simulink model "FOC_sensored"  (R2026a)
settings: Solver=VariableStepAuto  StopTime=3  MaxStep=1e-4  RelTol=1e-4
undefined symbols (not defined in the file): Encoder_resolution, G_filt_back_den_current, G_filt_back_num_current, G_filt_cont_den_current, G_filt_cont_num_current, G_filt_disc_emu_back_den_current, G_filt_disc_emu_back_num_current, G_filt_disc_emu_forw_den_current, G_filt_disc_emu_forw_num_current, G_filt_forw_den_current, G_filt_forw_num_current, In, J, Kr_cont_current, Kr_cont_speed, Kr_direct_back_current, Kr_direct_forw_current, Ld, Lq, Ls, Mn, nn, pp, Psir, T_speed_feedback, Ti_cont_current, Ti_cont_speed, Ti_direct_back_current, Ti_direct_forw_current, Ts_current, Udc
libraries: fl_lib x43, nesl_utility x37, ee_lib x18, eeTransforms x12, slpidlib x5
(part 2 of 2)

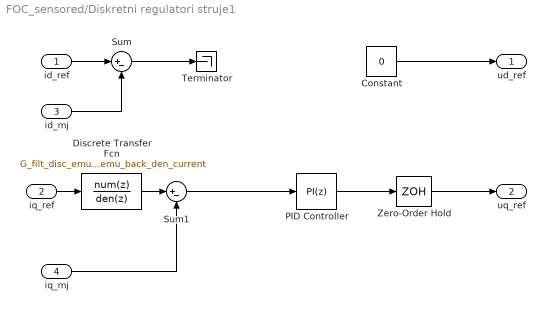
== system FOC_sensored/Diskretni regulatori struje1 ==
  id_ref : Inport
  iq_ref : Inport  Port=2
  id_mj : Inport  Port=3
  iq_mj : Inport  Port=4
  Constant : Constant  Value=0
  Discrete Transfer Fcn : DiscreteTransferFcn  Numerator=G_filt_disc_emu_back_num_current  Denominator=G_filt_disc_emu_back_den_current
  PID Controller : slpidlib/PID Controller  Controller=PI  Form=Ideal  TimeDomain=Discrete-time  UseExternalTs=off  SampleTime=-1  IntegratorMethod=Backward Euler  FilterMethod=Forward Euler  ControllerParametersSource=internal  P=Kr_cont_current  I=1/Ti_cont_current  UseKiTs=off  D=0  UseExternalDerivativeSource=off  N=100  UseFilter=on  TunerSelectOption=Transfer Function Based (PID Tuner App)  InitialConditionSource=internal  InitialConditionForIntegrator=0  InitialConditionForFilter=0  DifferentiatorICPrevScaledInput=0  ExternalReset=none  TrackingMode=off  Kt=1  LimitOutput=off  SatLimitsSource=internal  UpperSaturationLimit=inf  LowerSaturationLimit=-inf  LinearizeAsGain=on  AntiWindupMode=none  Kb=1  LimitIntegrator=off  UpperIntegratorSaturationLimit=inf  LowerIntegratorSaturationLimit=-inf  POutMin=[]  POutMax=[]  IOutMin=[]  IOutMax=[]  DOutMin=[]  DOutMax=[]  NOutMin=[]  NOutMax=[]  SumOutMin=[]  SumOutMax=[]  SaturationOutMin=[]  SaturationOutMax=[]  PParamMin=[]  PParamMax=[]  IParamMin=[]  IParamMax=[]  DParamMin=[]  DParamMax=[]  NParamMin=[]  NParamMax=[]  KbParamMin=[]  KbParamMax=[]  KtParamMin=[]  KtParamMax=[]  KbOutMin=[]  KbOutMax=[]  KtOutMin=[]  KtOutMax=[]  IntegratorOutMin=[]  IntegratorOutMax=[]  FilterOutMin=[]  FilterOutMax=[]  SumI1OutMin=[]  SumI1OutMax=[]  SumI2OutMin=[]  SumI2OutMax=[]  SumI3OutMin=[]  SumI3OutMax=[]  SumI4OutMin=[]  SumI4OutMax=[]  SumDOutMin=[]  SumDOutMax=[]  DifferentiatorOutMin=[]  DifferentiatorOutMax=[]  FilterDiffOutCoefMin=[]  FilterDiffOutCoefMax=[]  ReciprocalOutMin=[]  ReciprocalOutMax=[]  SumDenOutMin=[]  SumDenOutMax=[]  SumNumOutMin=[]  SumNumOutMax=[]  DivideOutMin=[]  DivideOutMax=[]  UdiffTsProdOutMin=[]  UdiffTsProdOutMax=[]  NTsProdOutMin=[]  NTsProdOutMax=[]  UintegralTsProdOutMin=[]  UintegralTsProdOutMax=[]  UngainTsProdOutMin=[]  UngainTsProdOutMax=[]  ClampingZeroOutDataTypeStr=Inherit: Inherit via back propagation  ClampingZeroOutMin=[]  ClampingZeroOutMax=[]  FilterDenConstantOutDataTypeStr=Inherit: Inherit via back propagation  FilterDenConstantOutMin=[]  FilterDenConstantOutMax=[]  PCopyOutDataTypeStr=Inherit: Inherit via back propagation  PCopyOutMin=[]  PCopyOutMax=[]  NCopyOutDataTypeStr=Inherit: Inherit via back propagation  NCopyOutMin=[]  NCopyOutMax=[]  IntegratorContinuousStateAttributes=''  IntegratorStateMustResolveToSignalObject=off  IntegratorRTWStateStorageClass=Auto  FilterContinuousStateAttributes=''  FilterStateMustResolveToSignalObject=off  FilterRTWStateStorageClass=Auto  ParallelPVariant=Passthrough  IdealPVariant=InternalParameters  IVariant=InternalParameters  DVariant=Disabled  IntegratorVariant=Discrete  SatVariant=Disabled  AWVariant=Passthrough  PCopyVariant=Disabled  TRVariant=Disabled  FdbkBlocksVariant=Forward  IdealPFdbkVariant=Disabled  SatFdbkVariant=Disabled  DerivativeFilterVariant=Disabled  NVariant=Disabled  NCopyVariant=Disabled_SignalSpec  FilterICVariant=Disabled  IntegratorICVariant=InternalICs  ExternalResetVariant=Disabled  TRSumVariant=Passthrough  SumFdbkVariant=Disabled  SumVariant=Sum_PI  TsampFilterVariant=InternalTs  TsampNgainVariant=Passthrough  TsampIntegralVariant=Disabled_SignalSpec  ExternalSaturationOutDataTypeStr=Inherit: Same as second input  DerivativeSourceVariant=Disabled  PreIntVariant=InternalPreInt
  Sum : Sum  Inputs=|+-
  Sum1 : Sum  Inputs=|+-
  Terminator : Terminator
  Zero-Order Hold : ZeroOrderHold  SampleTime=Ts_current
  ud_ref : Outport
  uq_ref : Outport  Port=2
  wires:
  iq_mj/1 -> Sum1/2
  Zero-Order Hold/1 -> uq_ref/1
  Sum1/1 -> PID Controller/1
  iq_ref/1 -> Discrete Transfer Fcn/1
  Discrete Transfer Fcn/1 -> Sum1/1
  PID Controller/1 -> Zero-Order Hold/1
  Sum/1 -> Terminator/1
  id_mj/1 -> Sum/2
  id_ref/1 -> Sum/1
  Constant/1 -> ud_ref/1

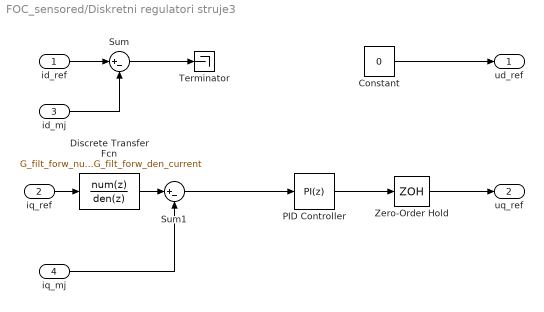
== system FOC_sensored/Diskretni regulatori struje3 ==
  id_ref : Inport
  iq_ref : Inport  Port=2
  id_mj : Inport  Port=3
  iq_mj : Inport  Port=4
  Constant : Constant  Value=0
  Discrete Transfer Fcn : DiscreteTransferFcn  Numerator=G_filt_forw_num_current  Denominator=G_filt_forw_den_current
  PID Controller : slpidlib/PID Controller  Controller=PI  Form=Ideal  TimeDomain=Discrete-time  UseExternalTs=off  SampleTime=-1  IntegratorMethod=Forward Euler  FilterMethod=Forward Euler  ControllerParametersSource=internal  P=Kr_direct_forw_current  I=1/Ti_direct_forw_current  UseKiTs=off  D=0  UseExternalDerivativeSource=off  N=100  UseFilter=on  TunerSelectOption=Transfer Function Based (PID Tuner App)  InitialConditionSource=internal  InitialConditionForIntegrator=0  InitialConditionForFilter=0  DifferentiatorICPrevScaledInput=0  ExternalReset=none  TrackingMode=off  Kt=1  LimitOutput=off  SatLimitsSource=internal  UpperSaturationLimit=inf  LowerSaturationLimit=-inf  LinearizeAsGain=on  AntiWindupMode=none  Kb=1  LimitIntegrator=off  UpperIntegratorSaturationLimit=inf  LowerIntegratorSaturationLimit=-inf  POutMin=[]  POutMax=[]  IOutMin=[]  IOutMax=[]  DOutMin=[]  DOutMax=[]  NOutMin=[]  NOutMax=[]  SumOutMin=[]  SumOutMax=[]  SaturationOutMin=[]  SaturationOutMax=[]  PParamMin=[]  PParamMax=[]  IParamMin=[]  IParamMax=[]  DParamMin=[]  DParamMax=[]  NParamMin=[]  NParamMax=[]  KbParamMin=[]  KbParamMax=[]  KtParamMin=[]  KtParamMax=[]  KbOutMin=[]  KbOutMax=[]  KtOutMin=[]  KtOutMax=[]  IntegratorOutMin=[]  IntegratorOutMax=[]  FilterOutMin=[]  FilterOutMax=[]  SumI1OutMin=[]  SumI1OutMax=[]  SumI2OutMin=[]  SumI2OutMax=[]  SumI3OutMin=[]  SumI3OutMax=[]  SumI4OutMin=[]  SumI4OutMax=[]  SumDOutMin=[]  SumDOutMax=[]  DifferentiatorOutMin=[]  DifferentiatorOutMax=[]  FilterDiffOutCoefMin=[]  FilterDiffOutCoefMax=[]  ReciprocalOutMin=[]  ReciprocalOutMax=[]  SumDenOutMin=[]  SumDenOutMax=[]  SumNumOutMin=[]  SumNumOutMax=[]  DivideOutMin=[]  DivideOutMax=[]  UdiffTsProdOutMin=[]  UdiffTsProdOutMax=[]  NTsProdOutMin=[]  NTsProdOutMax=[]  UintegralTsProdOutMin=[]  UintegralTsProdOutMax=[]  UngainTsProdOutMin=[]  UngainTsProdOutMax=[]  ClampingZeroOutDataTypeStr=Inherit: Inherit via back propagation  ClampingZeroOutMin=[]  ClampingZeroOutMax=[]  FilterDenConstantOutDataTypeStr=Inherit: Inherit via back propagation  FilterDenConstantOutMin=[]  FilterDenConstantOutMax=[]  PCopyOutDataTypeStr=Inherit: Inherit via back propagation  PCopyOutMin=[]  PCopyOutMax=[]  NCopyOutDataTypeStr=Inherit: Inherit via back propagation  NCopyOutMin=[]  NCopyOutMax=[]  IntegratorContinuousStateAttributes=''  IntegratorStateMustResolveToSignalObject=off  IntegratorRTWStateStorageClass=Auto  FilterContinuousStateAttributes=''  FilterStateMustResolveToSignalObject=off  FilterRTWStateStorageClass=Auto  ParallelPVariant=Passthrough  IdealPVariant=InternalParameters  IVariant=InternalParameters  DVariant=Disabled  IntegratorVariant=Discrete  SatVariant=Disabled  AWVariant=Passthrough  PCopyVariant=Disabled  TRVariant=Disabled  FdbkBlocksVariant=Forward  IdealPFdbkVariant=Disabled  SatFdbkVariant=Disabled  DerivativeFilterVariant=Disabled  NVariant=Disabled  NCopyVariant=Disabled_SignalSpec  FilterICVariant=Disabled  IntegratorICVariant=InternalICs  ExternalResetVariant=Disabled  TRSumVariant=Passthrough  SumFdbkVariant=Disabled  SumVariant=Sum_PI  TsampFilterVariant=InternalTs  TsampNgainVariant=Passthrough  TsampIntegralVariant=Disabled_SignalSpec  ExternalSaturationOutDataTypeStr=Inherit: Same as second input  DerivativeSourceVariant=Disabled  PreIntVariant=InternalPreInt
  Sum : Sum  Inputs=|+-
  Sum1 : Sum  Inputs=|+-
  Terminator : Terminator
  Zero-Order Hold : ZeroOrderHold  SampleTime=Ts_current
  ud_ref : Outport
  uq_ref : Outport  Port=2
  wires:
  iq_mj/1 -> Sum1/2
  Zero-Order Hold/1 -> uq_ref/1
  Sum1/1 -> PID Controller/1
  iq_ref/1 -> Discrete Transfer Fcn/1
  Discrete Transfer Fcn/1 -> Sum1/1
  PID Controller/1 -> Zero-Order Hold/1
  Sum/1 -> Terminator/1
  id_mj/1 -> Sum/2
  id_ref/1 -> Sum/1
  Constant/1 -> ud_ref/1

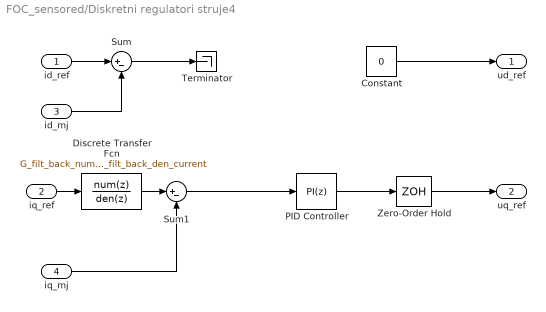
== system FOC_sensored/Diskretni regulatori struje4 ==
  id_ref : Inport
  iq_ref : Inport  Port=2
  id_mj : Inport  Port=3
  iq_mj : Inport  Port=4
  Constant : Constant  Value=0
  Discrete Transfer Fcn : DiscreteTransferFcn  Numerator=G_filt_back_num_current  Denominator=G_filt_back_den_current
  PID Controller : slpidlib/PID Controller  Controller=PI  Form=Ideal  TimeDomain=Discrete-time  UseExternalTs=off  SampleTime=-1  IntegratorMethod=Backward Euler  FilterMethod=Forward Euler  ControllerParametersSource=internal  P=Kr_direct_back_current  I=1/Ti_direct_back_current  UseKiTs=off  D=0  UseExternalDerivativeSource=off  N=100  UseFilter=on  TunerSelectOption=Transfer Function Based (PID Tuner App)  InitialConditionSource=internal  InitialConditionForIntegrator=0  InitialConditionForFilter=0  DifferentiatorICPrevScaledInput=0  ExternalReset=none  TrackingMode=off  Kt=1  LimitOutput=off  SatLimitsSource=internal  UpperSaturationLimit=inf  LowerSaturationLimit=-inf  LinearizeAsGain=on  AntiWindupMode=none  Kb=1  LimitIntegrator=off  UpperIntegratorSaturationLimit=inf  LowerIntegratorSaturationLimit=-inf  POutMin=[]  POutMax=[]  IOutMin=[]  IOutMax=[]  DOutMin=[]  DOutMax=[]  NOutMin=[]  NOutMax=[]  SumOutMin=[]  SumOutMax=[]  SaturationOutMin=[]  SaturationOutMax=[]  PParamMin=[]  PParamMax=[]  IParamMin=[]  IParamMax=[]  DParamMin=[]  DParamMax=[]  NParamMin=[]  NParamMax=[]  KbParamMin=[]  KbParamMax=[]  KtParamMin=[]  KtParamMax=[]  KbOutMin=[]  KbOutMax=[]  KtOutMin=[]  KtOutMax=[]  IntegratorOutMin=[]  IntegratorOutMax=[]  FilterOutMin=[]  FilterOutMax=[]  SumI1OutMin=[]  SumI1OutMax=[]  SumI2OutMin=[]  SumI2OutMax=[]  SumI3OutMin=[]  SumI3OutMax=[]  SumI4OutMin=[]  SumI4OutMax=[]  SumDOutMin=[]  SumDOutMax=[]  DifferentiatorOutMin=[]  DifferentiatorOutMax=[]  FilterDiffOutCoefMin=[]  FilterDiffOutCoefMax=[]  ReciprocalOutMin=[]  ReciprocalOutMax=[]  SumDenOutMin=[]  SumDenOutMax=[]  SumNumOutMin=[]  SumNumOutMax=[]  DivideOutMin=[]  DivideOutMax=[]  UdiffTsProdOutMin=[]  UdiffTsProdOutMax=[]  NTsProdOutMin=[]  NTsProdOutMax=[]  UintegralTsProdOutMin=[]  UintegralTsProdOutMax=[]  UngainTsProdOutMin=[]  UngainTsProdOutMax=[]  ClampingZeroOutDataTypeStr=Inherit: Inherit via back propagation  ClampingZeroOutMin=[]  ClampingZeroOutMax=[]  FilterDenConstantOutDataTypeStr=Inherit: Inherit via back propagation  FilterDenConstantOutMin=[]  FilterDenConstantOutMax=[]  PCopyOutDataTypeStr=Inherit: Inherit via back propagation  PCopyOutMin=[]  PCopyOutMax=[]  NCopyOutDataTypeStr=Inherit: Inherit via back propagation  NCopyOutMin=[]  NCopyOutMax=[]  IntegratorContinuousStateAttributes=''  IntegratorStateMustResolveToSignalObject=off  IntegratorRTWStateStorageClass=Auto  FilterContinuousStateAttributes=''  FilterStateMustResolveToSignalObject=off  FilterRTWStateStorageClass=Auto  ParallelPVariant=Passthrough  IdealPVariant=InternalParameters  IVariant=InternalParameters  DVariant=Disabled  IntegratorVariant=Discrete  SatVariant=Disabled  AWVariant=Passthrough  PCopyVariant=Disabled  TRVariant=Disabled  FdbkBlocksVariant=Forward  IdealPFdbkVariant=Disabled  SatFdbkVariant=Disabled  DerivativeFilterVariant=Disabled  NVariant=Disabled  NCopyVariant=Disabled_SignalSpec  FilterICVariant=Disabled  IntegratorICVariant=InternalICs  ExternalResetVariant=Disabled  TRSumVariant=Passthrough  SumFdbkVariant=Disabled  SumVariant=Sum_PI  TsampFilterVariant=InternalTs  TsampNgainVariant=Passthrough  TsampIntegralVariant=Disabled_SignalSpec  ExternalSaturationOutDataTypeStr=Inherit: Same as second input  DerivativeSourceVariant=Disabled  PreIntVariant=InternalPreInt
  Sum : Sum  Inputs=|+-
  Sum1 : Sum  Inputs=|+-
  Terminator : Terminator
  Zero-Order Hold : ZeroOrderHold  SampleTime=Ts_current
  ud_ref : Outport
  uq_ref : Outport  Port=2
  wires:
  Sum/1 -> Terminator/1
  id_ref/1 -> Sum/1
  Constant/1 -> ud_ref/1
  Sum1/1 -> PID Controller/1
  id_mj/1 -> Sum/2
  iq_mj/1 -> Sum1/2
  Zero-Order Hold/1 -> uq_ref/1
  PID Controller/1 -> Zero-Order Hold/1
  iq_ref/1 -> Discrete Transfer Fcn/1
  Discrete Transfer Fcn/1 -> Sum1/1

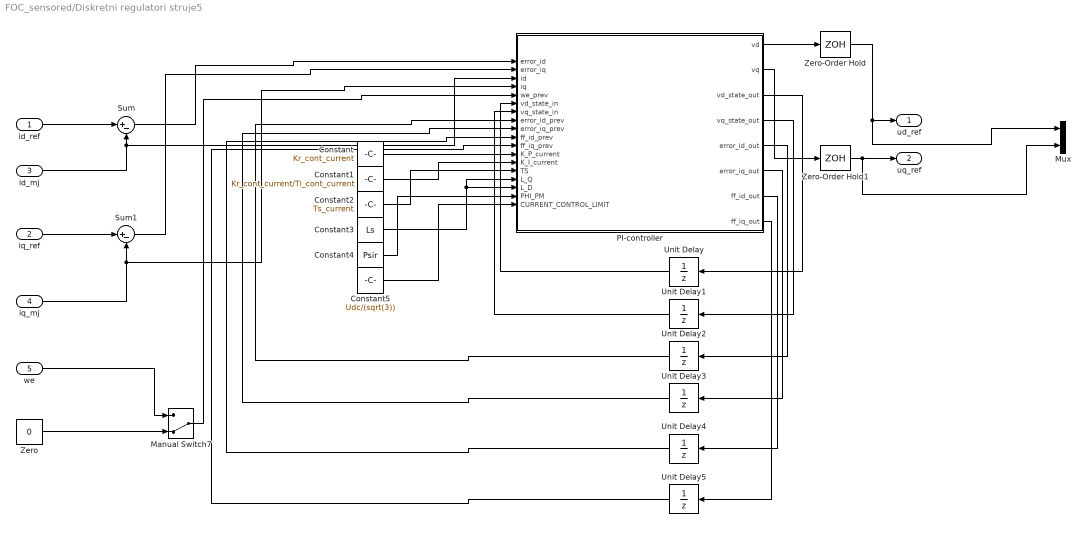
== system FOC_sensored/Diskretni regulatori struje5 ==
  id_ref : Inport
  iq_ref : Inport  Port=2
  id_mj : Inport  Port=3
  iq_mj : Inport  Port=4
  we : Inport  Port=5
  Constant : Constant  Value=Kr_cont_current  SampleTime=Ts_current
  Constant1 : Constant  Value=Kr_cont_current/Ti_cont_current  SampleTime=Ts_current
  Constant2 : Constant  Value=Ts_current  SampleTime=Ts_current
  Constant3 : Constant  Value=Ls  SampleTime=Ts_current
  Constant4 : Constant  Value=Psir  SampleTime=Ts_current
  Constant5 : Constant  Value=Udc/(sqrt(3))  SampleTime=Ts_current
  Manual Switch7 : ManualSwitch  CurrentSetting=0
  Mux : Mux  Inputs=2
  PI-controller : MATLAB Function  TreatAsAtomicUnit=on
  Sum : Sum  Inputs=|+-
  Sum1 : Sum  Inputs=|+-
  Unit Delay{,1..5} (6 alike) : UnitDelay  SampleTime=Ts_current
  Zero : Constant  Value=0  OutDataTypeStr=Inherit: Inherit via back propagation
  Zero-Order Hold : ZeroOrderHold  SampleTime=Ts_current
  Zero-Order Hold1 : ZeroOrderHold  SampleTime=Ts_current
  ud_ref : Outport
  uq_ref : Outport  Port=2
  wires:
  id_ref/1 -> Sum/1
  iq_ref/1 -> Sum1/1
  Sum/1 -> PI-controller/1(error_id)
  Sum1/1 -> PI-controller/2(error_iq)
  id_mj/1 -> Sum/2, PI-controller/3(id)
  iq_mj/1 -> PI-controller/4(iq), Sum1/2
  PI-controller/3(vd_state_out) -> Unit Delay/1
  PI-controller/4(vq_state_out) -> Unit Delay1/1
  PI-controller/5(error_id_out) -> Unit Delay2/1
  PI-controller/6(error_iq_out) -> Unit Delay3/1
  Unit Delay/1 -> PI-controller/6(vd_state_in)
  Unit Delay1/1 -> PI-controller/7(vq_state_in)
  Unit Delay2/1 -> PI-controller/8(error_id_prev)
  Unit Delay3/1 -> PI-controller/9(error_iq_prev)
  PI-controller/1(vd) -> Zero-Order Hold/1
  PI-controller/2(vq) -> Zero-Order Hold1/1
  Zero-Order Hold/1 -> Mux/1, ud_ref/1
  Zero-Order Hold1/1 -> Mux/2, uq_ref/1
  PI-controller/7(ff_id_out) -> Unit Delay4/1
  PI-controller/8(ff_iq_out) -> Unit Delay5/1
  Unit Delay4/1 -> PI-controller/10(ff_id_prev)
  Unit Delay5/1 -> PI-controller/11(ff_iq_prev)
  Zero/1 -> Manual Switch7/2
  Manual Switch7/1 -> PI-controller/5(we_prev)
  we/1 -> Manual Switch7/1
  Constant/1 -> PI-controller/12(K_P_current)
  Constant1/1 -> PI-controller/13(K_I_current)
  Constant2/1 -> PI-controller/14(TS)
  Constant3/1 -> PI-controller/16(L_D), PI-controller/15(L_Q)
  Constant4/1 -> PI-controller/17(PHI_PM)
  Constant5/1 -> PI-controller/18(CURRENT_CONTROL_LIMIT)

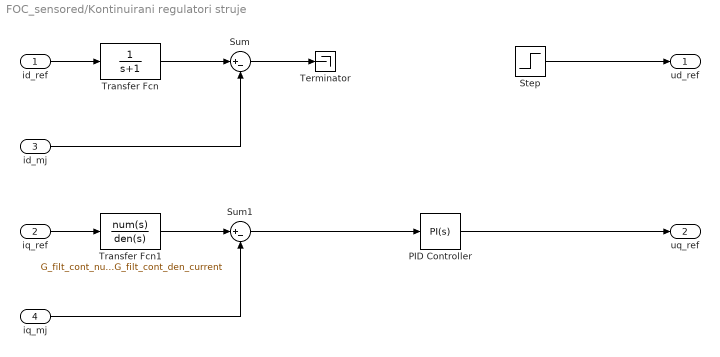
== system FOC_sensored/Kontinuirani regulatori struje ==
  id_ref : Inport
  iq_ref : Inport  Port=2
  id_mj : Inport  Port=3
  iq_mj : Inport  Port=4
  PID Controller : slpidlib/PID Controller  Controller=PI  Form=Ideal  TimeDomain=Continuous-time  UseExternalTs=off  SampleTime=-1  IntegratorMethod=Forward Euler  FilterMethod=Forward Euler  ControllerParametersSource=internal  P=Kr_cont_current  I=1/Ti_cont_current  UseKiTs=off  D=0  UseExternalDerivativeSource=off  N=100  UseFilter=on  TunerSelectOption=Transfer Function Based (PID Tuner App)  InitialConditionSource=internal  InitialConditionForIntegrator=0  InitialConditionForFilter=0  DifferentiatorICPrevScaledInput=0  ExternalReset=none  TrackingMode=off  Kt=1  LimitOutput=off  SatLimitsSource=internal  UpperSaturationLimit=inf  LowerSaturationLimit=-inf  LinearizeAsGain=on  AntiWindupMode=none  Kb=1  LimitIntegrator=off  UpperIntegratorSaturationLimit=inf  LowerIntegratorSaturationLimit=-inf  POutMin=[]  POutMax=[]  IOutMin=[]  IOutMax=[]  DOutMin=[]  DOutMax=[]  NOutMin=[]  NOutMax=[]  SumOutMin=[]  SumOutMax=[]  SaturationOutMin=[]  SaturationOutMax=[]  PParamMin=[]  PParamMax=[]  IParamMin=[]  IParamMax=[]  DParamMin=[]  DParamMax=[]  NParamMin=[]  NParamMax=[]  KbParamMin=[]  KbParamMax=[]  KtParamMin=[]  KtParamMax=[]  KbOutMin=[]  KbOutMax=[]  KtOutMin=[]  KtOutMax=[]  IntegratorOutMin=[]  IntegratorOutMax=[]  FilterOutMin=[]  FilterOutMax=[]  SumI1OutMin=[]  SumI1OutMax=[]  SumI2OutMin=[]  SumI2OutMax=[]  SumI3OutMin=[]  SumI3OutMax=[]  SumI4OutMin=[]  SumI4OutMax=[]  SumDOutMin=[]  SumDOutMax=[]  DifferentiatorOutMin=[]  DifferentiatorOutMax=[]  FilterDiffOutCoefMin=[]  FilterDiffOutCoefMax=[]  ReciprocalOutMin=[]  ReciprocalOutMax=[]  SumDenOutMin=[]  SumDenOutMax=[]  SumNumOutMin=[]  SumNumOutMax=[]  DivideOutMin=[]  DivideOutMax=[]  UdiffTsProdOutMin=[]  UdiffTsProdOutMax=[]  NTsProdOutMin=[]  NTsProdOutMax=[]  UintegralTsProdOutMin=[]  UintegralTsProdOutMax=[]  UngainTsProdOutMin=[]  UngainTsProdOutMax=[]  ClampingZeroOutDataTypeStr=Inherit: Inherit via back propagation  ClampingZeroOutMin=[]  ClampingZeroOutMax=[]  FilterDenConstantOutDataTypeStr=Inherit: Inherit via back propagation  FilterDenConstantOutMin=[]  FilterDenConstantOutMax=[]  PCopyOutDataTypeStr=Inherit: Inherit via back propagation  PCopyOutMin=[]  PCopyOutMax=[]  NCopyOutDataTypeStr=Inherit: Inherit via back propagation  NCopyOutMin=[]  NCopyOutMax=[]  IntegratorContinuousStateAttributes=''  IntegratorStateMustResolveToSignalObject=off  IntegratorRTWStateStorageClass=Auto  FilterContinuousStateAttributes=''  FilterStateMustResolveToSignalObject=off  FilterRTWStateStorageClass=Auto  ParallelPVariant=Passthrough  IdealPVariant=InternalParameters  IVariant=InternalParameters  DVariant=Disabled  IntegratorVariant=Continuous  SatVariant=Disabled  AWVariant=Passthrough  PCopyVariant=Disabled  TRVariant=Disabled  FdbkBlocksVariant=Forward  IdealPFdbkVariant=Disabled  SatFdbkVariant=Disabled  DerivativeFilterVariant=Disabled  NVariant=Disabled  NCopyVariant=Disabled_SignalSpec  FilterICVariant=Disabled  IntegratorICVariant=InternalICs  ExternalResetVariant=Disabled  TRSumVariant=Passthrough  SumFdbkVariant=Disabled  SumVariant=Sum_PI  TsampFilterVariant=InternalTs  TsampNgainVariant=Passthrough  TsampIntegralVariant=Disabled_SignalSpec  ExternalSaturationOutDataTypeStr=Inherit: Same as second input  DerivativeSourceVariant=Disabled  PreIntVariant=InternalPreInt
  Step : Step  FinalValue=0  SampleTime=0
  Sum : Sum  Inputs=|+-
  Sum1 : Sum  Inputs=|+-
  Terminator : Terminator
  Transfer Fcn : TransferFcn  Denominator=[1 1]
  Transfer Fcn1 : TransferFcn  Numerator=G_filt_cont_num_current  Denominator=G_filt_cont_den_current
  ud_ref : Outport
  uq_ref : Outport  Port=2
  wires:
  id_ref/1 -> Transfer Fcn/1
  Transfer Fcn/1 -> Sum/1
  id_mj/1 -> Sum/2
  iq_ref/1 -> Transfer Fcn1/1
  Transfer Fcn1/1 -> Sum1/1
  iq_mj/1 -> Sum1/2
  Sum1/1 -> PID Controller/1
  PID Controller/1 -> uq_ref/1
  Sum/1 -> Terminator/1
  Step/1 -> ud_ref/1

== system FOC_sensored/Mjerenje momenta ==
  PS-Simulink Converter3 : nesl_utility/PS-Simulink Converter  PhysicalDomain=network_engine_domain  SubClassName=ps_output  LeftPortType=input  RightPortType=output  PseudoPeriodic=off  Frequencies=[]  VectorFormat=1-D array  Unit=N*m  AffineConversion=off
  Torque Sensor : fl_lib/Mechanical/Mechanical Sensors/Ideal Torque Sensor
  R : PMIOPort  Side=Left
  C : PMIOPort  Port=2  Side=Right
  Output : Outport
  wires:
  PS-Simulink Converter3/1 -> Output/1
  connections:
  Torque Sensor/RConn1 -- C/RConn1
  Torque Sensor/RConn2 -- PS-Simulink Converter3/LConn1
  Torque Sensor/LConn1 -- R/RConn1

== system FOC_sensored/Mjerenje momenta1 ==
  PS-Simulink Converter3 : nesl_utility/PS-Simulink Converter  PhysicalDomain=network_engine_domain  SubClassName=ps_output  LeftPortType=input  RightPortType=output  PseudoPeriodic=off  Frequencies=[]  VectorFormat=1-D array  Unit=N*m  AffineConversion=off
  Torque Sensor : fl_lib/Mechanical/Mechanical Sensors/Ideal Torque Sensor
  R : PMIOPort  Side=Left
  C : PMIOPort  Port=2  Side=Right
  Output : Outport
  wires:
  PS-Simulink Converter3/1 -> Output/1
  connections:
  Torque Sensor/RConn1 -- C/RConn1
  Torque Sensor/RConn2 -- PS-Simulink Converter3/LConn1
  Torque Sensor/LConn1 -- R/RConn1

== system FOC_sensored/Mjerenje momenta2 ==
  PS-Simulink Converter3 : nesl_utility/PS-Simulink Converter  PhysicalDomain=network_engine_domain  SubClassName=ps_output  LeftPortType=input  RightPortType=output  PseudoPeriodic=off  Frequencies=[]  VectorFormat=1-D array  Unit=N*m  AffineConversion=off
  Torque Sensor : fl_lib/Mechanical/Mechanical Sensors/Ideal Torque Sensor
  R : PMIOPort  Side=Left
  C : PMIOPort  Port=2  Side=Right
  Output : Outport
  wires:
  PS-Simulink Converter3/1 -> Output/1
  connections:
  Torque Sensor/RConn1 -- C/RConn1
  Torque Sensor/RConn2 -- PS-Simulink Converter3/LConn1
  Torque Sensor/LConn1 -- R/RConn1

== system FOC_sensored/Mjerenje momenta4 ==
  PS-Simulink Converter3 : nesl_utility/PS-Simulink Converter  PhysicalDomain=network_engine_domain  SubClassName=ps_output  LeftPortType=input  RightPortType=output  PseudoPeriodic=off  Frequencies=[]  VectorFormat=1-D array  Unit=N*m  AffineConversion=off
  Torque Sensor : fl_lib/Mechanical/Mechanical Sensors/Ideal Torque Sensor
  R : PMIOPort  Side=Left
  C : PMIOPort  Port=2  Side=Right
  Output : Outport
  wires:
  PS-Simulink Converter3/1 -> Output/1
  connections:
  Torque Sensor/RConn1 -- C/RConn1
  Torque Sensor/RConn2 -- PS-Simulink Converter3/LConn1
  Torque Sensor/LConn1 -- R/RConn1

== system FOC_sensored/Mjerenje momenta5 ==
  PS-Simulink Converter3 : nesl_utility/PS-Simulink Converter  PhysicalDomain=network_engine_domain  SubClassName=ps_output  LeftPortType=input  RightPortType=output  PseudoPeriodic=off  Frequencies=[]  VectorFormat=1-D array  Unit=N*m  AffineConversion=off
  Torque Sensor : fl_lib/Mechanical/Mechanical Sensors/Ideal Torque Sensor
  R : PMIOPort  Side=Left
  C : PMIOPort  Port=2  Side=Right
  Output : Outport
  wires:
  PS-Simulink Converter3/1 -> Output/1
  connections:
  Torque Sensor/RConn1 -- C/RConn1
  Torque Sensor/RConn2 -- PS-Simulink Converter3/LConn1
  Torque Sensor/LConn1 -- R/RConn1

== system FOC_sensored/Mjerenje momenta6 ==
  PS-Simulink Converter3 : nesl_utility/PS-Simulink Converter  PhysicalDomain=network_engine_domain  SubClassName=ps_output  LeftPortType=input  RightPortType=output  PseudoPeriodic=off  Frequencies=[]  VectorFormat=1-D array  Unit=N*m  AffineConversion=off
  Torque Sensor : fl_lib/Mechanical/Mechanical Sensors/Ideal Torque Sensor
  R : PMIOPort  Side=Left
  C : PMIOPort  Port=2  Side=Right
  Output : Outport
  wires:
  PS-Simulink Converter3/1 -> Output/1
  connections:
  Torque Sensor/RConn1 -- C/RConn1
  Torque Sensor/RConn2 -- PS-Simulink Converter3/LConn1
  Torque Sensor/LConn1 -- R/RConn1

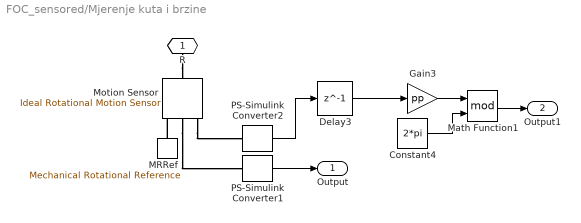
== system FOC_sensored/Mjerenje kuta i brzine ==
  Constant4 : Constant  Value=2*pi
  Delay3 : Delay  DelayLength=1  SampleTime=Ts_current
  Gain3 : Gain  Gain=pp
  MRRef : fl_lib/Mechanical/Rotational Elements/Mechanical Rotational Reference
  Math Function1 : Math  Operator=mod
  Motion Sensor : fl_lib/Mechanical/Mechanical Sensors/Ideal Rotational Motion Sensor  reference=foundation.enum.MeasurementReference.difference  acceleration_port=false  velocity_port=true  position_port=true  wrap_angle=simscape.enum.onoff.off  offset=0 deg
  PS-Simulink Converter1 : nesl_utility/PS-Simulink Converter  PhysicalDomain=network_engine_domain  SubClassName=ps_output  LeftPortType=input  RightPortType=output  PseudoPeriodic=off  Frequencies=[]  VectorFormat=1-D array  Unit=rad/s  AffineConversion=off
  PS-Simulink Converter2 : nesl_utility/PS-Simulink Converter  PhysicalDomain=network_engine_domain  SubClassName=ps_output  LeftPortType=input  RightPortType=output  PseudoPeriodic=off  Frequencies=[]  VectorFormat=1-D array  Unit=rad  AffineConversion=off
  R : PMIOPort  Side=Left
  Output : Outport
  Output1 : Outport  Port=2
  wires:
  PS-Simulink Converter1/1 -> Output/1
  Gain3/1 -> Math Function1/1
  Delay3/1 -> Gain3/1
  Constant4/1 -> Math Function1/2
  Math Function1/1 -> Output1/1
  PS-Simulink Converter2/1 -> Delay3/1
  connections:
  R/RConn1 -- Motion Sensor/LConn1
  Motion Sensor/RConn2 -- PS-Simulink Converter1/LConn1
  MRRef/LConn1 -- Motion Sensor/RConn1
  Motion Sensor/RConn3 -- PS-Simulink Converter2/LConn1

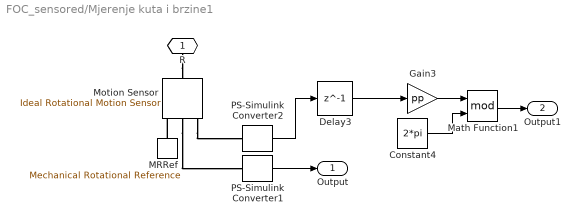
== system FOC_sensored/Mjerenje kuta i brzine1 ==
  Constant4 : Constant  Value=2*pi
  Delay3 : Delay  DelayLength=1  SampleTime=Ts_current
  Gain3 : Gain  Gain=pp
  MRRef : fl_lib/Mechanical/Rotational Elements/Mechanical Rotational Reference
  Math Function1 : Math  Operator=mod
  Motion Sensor : fl_lib/Mechanical/Mechanical Sensors/Ideal Rotational Motion Sensor  reference=foundation.enum.MeasurementReference.difference  acceleration_port=false  velocity_port=true  position_port=true  wrap_angle=simscape.enum.onoff.off  offset=0 deg
  PS-Simulink Converter1 : nesl_utility/PS-Simulink Converter  PhysicalDomain=network_engine_domain  SubClassName=ps_output  LeftPortType=input  RightPortType=output  PseudoPeriodic=off  Frequencies=[]  VectorFormat=1-D array  Unit=rad/s  AffineConversion=off
  PS-Simulink Converter2 : nesl_utility/PS-Simulink Converter  PhysicalDomain=network_engine_domain  SubClassName=ps_output  LeftPortType=input  RightPortType=output  PseudoPeriodic=off  Frequencies=[]  VectorFormat=1-D array  Unit=rad  AffineConversion=off
  R : PMIOPort  Side=Left
  Output : Outport
  Output1 : Outport  Port=2
  wires:
  PS-Simulink Converter1/1 -> Output/1
  Gain3/1 -> Math Function1/1
  Delay3/1 -> Gain3/1
  Constant4/1 -> Math Function1/2
  Math Function1/1 -> Output1/1
  PS-Simulink Converter2/1 -> Delay3/1
  connections:
  R/RConn1 -- Motion Sensor/LConn1
  Motion Sensor/RConn2 -- PS-Simulink Converter1/LConn1
  MRRef/LConn1 -- Motion Sensor/RConn1
  Motion Sensor/RConn3 -- PS-Simulink Converter2/LConn1

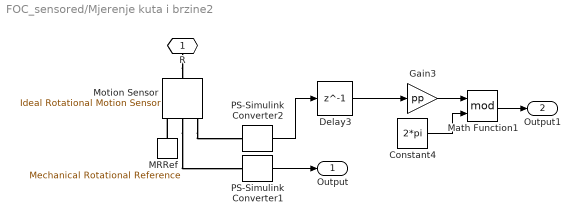
== system FOC_sensored/Mjerenje kuta i brzine2 ==
  Constant4 : Constant  Value=2*pi
  Delay3 : Delay  DelayLength=1  SampleTime=Ts_current
  Gain3 : Gain  Gain=pp
  MRRef : fl_lib/Mechanical/Rotational Elements/Mechanical Rotational Reference
  Math Function1 : Math  Operator=mod
  Motion Sensor : fl_lib/Mechanical/Mechanical Sensors/Ideal Rotational Motion Sensor  reference=foundation.enum.MeasurementReference.difference  acceleration_port=false  velocity_port=true  position_port=true  wrap_angle=simscape.enum.onoff.off  offset=0 deg
  PS-Simulink Converter1 : nesl_utility/PS-Simulink Converter  PhysicalDomain=network_engine_domain  SubClassName=ps_output  LeftPortType=input  RightPortType=output  PseudoPeriodic=off  Frequencies=[]  VectorFormat=1-D array  Unit=rad/s  AffineConversion=off
  PS-Simulink Converter2 : nesl_utility/PS-Simulink Converter  PhysicalDomain=network_engine_domain  SubClassName=ps_output  LeftPortType=input  RightPortType=output  PseudoPeriodic=off  Frequencies=[]  VectorFormat=1-D array  Unit=rad  AffineConversion=off
  R : PMIOPort  Side=Left
  Output : Outport
  Output1 : Outport  Port=2
  wires:
  PS-Simulink Converter1/1 -> Output/1
  Gain3/1 -> Math Function1/1
  Delay3/1 -> Gain3/1
  Constant4/1 -> Math Function1/2
  Math Function1/1 -> Output1/1
  PS-Simulink Converter2/1 -> Delay3/1
  connections:
  R/RConn1 -- Motion Sensor/LConn1
  Motion Sensor/RConn2 -- PS-Simulink Converter1/LConn1
  MRRef/LConn1 -- Motion Sensor/RConn1
  Motion Sensor/RConn3 -- PS-Simulink Converter2/LConn1

== system FOC_sensored/Mjerenje kuta i brzine4 ==
  Constant4 : Constant  Value=2*pi
  Delay3 : Delay  DelayLength=1  SampleTime=Ts_current
  Gain3 : Gain  Gain=pp
  MRRef : fl_lib/Mechanical/Rotational Elements/Mechanical Rotational Reference
  Math Function1 : Math  Operator=mod
  Motion Sensor : fl_lib/Mechanical/Mechanical Sensors/Ideal Rotational Motion Sensor  reference=foundation.enum.MeasurementReference.difference  acceleration_port=false  velocity_port=true  position_port=true  wrap_angle=simscape.enum.onoff.off  offset=0 deg
  PS-Simulink Converter1 : nesl_utility/PS-Simulink Converter  PhysicalDomain=network_engine_domain  SubClassName=ps_output  LeftPortType=input  RightPortType=output  PseudoPeriodic=off  Frequencies=[]  VectorFormat=1-D array  Unit=rad/s  AffineConversion=off
  PS-Simulink Converter2 : nesl_utility/PS-Simulink Converter  PhysicalDomain=network_engine_domain  SubClassName=ps_output  LeftPortType=input  RightPortType=output  PseudoPeriodic=off  Frequencies=[]  VectorFormat=1-D array  Unit=rad  AffineConversion=off
  R : PMIOPort  Side=Left
  Output : Outport
  Output1 : Outport  Port=2
  wires:
  PS-Simulink Converter1/1 -> Output/1
  Gain3/1 -> Math Function1/1
  Delay3/1 -> Gain3/1
  Constant4/1 -> Math Function1/2
  Math Function1/1 -> Output1/1
  PS-Simulink Converter2/1 -> Delay3/1
  connections:
  R/RConn1 -- Motion Sensor/LConn1
  Motion Sensor/RConn2 -- PS-Simulink Converter1/LConn1
  MRRef/LConn1 -- Motion Sensor/RConn1
  Motion Sensor/RConn3 -- PS-Simulink Converter2/LConn1

== system FOC_sensored/Mjerenje kuta i brzine5 ==
  Constant4 : Constant  Value=2*pi
  Delay3 : Delay  DelayLength=1  SampleTime=Ts_current
  Gain3 : Gain  Gain=pp
  MRRef : fl_lib/Mechanical/Rotational Elements/Mechanical Rotational Reference
  Math Function1 : Math  Operator=mod
  Motion Sensor : fl_lib/Mechanical/Mechanical Sensors/Ideal Rotational Motion Sensor  reference=foundation.enum.MeasurementReference.difference  acceleration_port=false  velocity_port=true  position_port=true  wrap_angle=simscape.enum.onoff.off  offset=0 deg
  PS-Simulink Converter1 : nesl_utility/PS-Simulink Converter  PhysicalDomain=network_engine_domain  SubClassName=ps_output  LeftPortType=input  RightPortType=output  PseudoPeriodic=off  Frequencies=[]  VectorFormat=1-D array  Unit=rad/s  AffineConversion=off
  PS-Simulink Converter2 : nesl_utility/PS-Simulink Converter  PhysicalDomain=network_engine_domain  SubClassName=ps_output  LeftPortType=input  RightPortType=output  PseudoPeriodic=off  Frequencies=[]  VectorFormat=1-D array  Unit=rad  AffineConversion=off
  R : PMIOPort  Side=Left
  Output : Outport
  Output1 : Outport  Port=2
  wires:
  PS-Simulink Converter1/1 -> Output/1
  Gain3/1 -> Math Function1/1
  Delay3/1 -> Gain3/1
  Constant4/1 -> Math Function1/2
  Math Function1/1 -> Output1/1
  PS-Simulink Converter2/1 -> Delay3/1
  connections:
  R/RConn1 -- Motion Sensor/LConn1
  Motion Sensor/RConn2 -- PS-Simulink Converter1/LConn1
  MRRef/LConn1 -- Motion Sensor/RConn1
  Motion Sensor/RConn3 -- PS-Simulink Converter2/LConn1

== system FOC_sensored/Mjerenje kuta i brzine6 ==
  Constant4 : Constant  Value=2*pi
  Gain : Gain  Gain=pp
  Gain3 : Gain  Gain=pp
  MRRef : fl_lib/Mechanical/Rotational Elements/Mechanical Rotational Reference
  Math Function1 : Math  Operator=mod
  Motion Sensor : fl_lib/Mechanical/Mechanical Sensors/Ideal Rotational Motion Sensor  reference=foundation.enum.MeasurementReference.difference  acceleration_port=false  velocity_port=true  position_port=true  wrap_angle=simscape.enum.onoff.off  offset=0 deg
  PS-Simulink Converter1 : nesl_utility/PS-Simulink Converter  PhysicalDomain=network_engine_domain  SubClassName=ps_output  LeftPortType=input  RightPortType=output  PseudoPeriodic=off  Frequencies=[]  VectorFormat=1-D array  Unit=rad/s  AffineConversion=off
  PS-Simulink Converter2 : nesl_utility/PS-Simulink Converter  PhysicalDomain=network_engine_domain  SubClassName=ps_output  LeftPortType=input  RightPortType=output  PseudoPeriodic=off  Frequencies=[]  VectorFormat=1-D array  Unit=rad  AffineConversion=off
  R : PMIOPort  Side=Left
  we : Outport
  theta_e : Outport  Port=2
  wires:
  PS-Simulink Converter1/1 -> Gain/1
  Gain/1 -> we/1
  PS-Simulink Converter2/1 -> Gain3/1
  Constant4/1 -> Math Function1/2
  Gain3/1 -> Math Function1/1
  Math Function1/1 -> theta_e/1
  connections:
  R/RConn1 -- Motion Sensor/LConn1
  Motion Sensor/RConn2 -- PS-Simulink Converter1/LConn1
  MRRef/LConn1 -- Motion Sensor/RConn1
  Motion Sensor/RConn3 -- PS-Simulink Converter2/LConn1

== system FOC_sensored/Mjerenje struje ==
  Input : Inport
  Current Sensor : ee_lib/Sensors & Transducers/Current Sensor (Three-Phase)  port_option=ee.enum.threePhasePort.composite
  PS-Simulink Converter : nesl_utility/PS-Simulink Converter  PhysicalDomain=network_engine_domain  SubClassName=ps_output  LeftPortType=input  RightPortType=output  PseudoPeriodic=off  Frequencies=[]  VectorFormat=1-D array  Unit=1  AffineConversion=off
  Park Transform : eeTransforms/Park Transform  AxisAlignment=D-axis  PowerInvariant=off
  ~1 : PMIOPort  Side=Left
  ~2 : PMIOPort  Port=2  Side=Right
  Output : Outport
  wires:
  PS-Simulink Converter/1 -> Park Transform/1
  Park Transform/1 -> Output/1
  Input/1 -> Park Transform/2
  connections:
  Current Sensor/LConn1 -- ~1/RConn1
  PS-Simulink Converter/LConn1 -- Current Sensor/RConn1
  Current Sensor/RConn2 -- ~2/RConn1

== system FOC_sensored/Mjerenje struje1 ==
  Input : Inport
  Current Sensor : ee_lib/Sensors & Transducers/Current Sensor (Three-Phase)  port_option=ee.enum.threePhasePort.composite
  PS-Simulink Converter : nesl_utility/PS-Simulink Converter  PhysicalDomain=network_engine_domain  SubClassName=ps_output  LeftPortType=input  RightPortType=output  PseudoPeriodic=off  Frequencies=[]  VectorFormat=1-D array  Unit=1  AffineConversion=off
  Park Transform : eeTransforms/Park Transform  AxisAlignment=D-axis  PowerInvariant=off
  ~1 : PMIOPort  Side=Left
  ~2 : PMIOPort  Port=2  Side=Right
  Output : Outport
  wires:
  PS-Simulink Converter/1 -> Park Transform/1
  Park Transform/1 -> Output/1
  Input/1 -> Park Transform/2
  connections:
  Current Sensor/LConn1 -- ~1/RConn1
  PS-Simulink Converter/LConn1 -- Current Sensor/RConn1
  Current Sensor/RConn2 -- ~2/RConn1

== system FOC_sensored/Mjerenje struje3 ==
  Input : Inport
  Current Sensor : ee_lib/Sensors & Transducers/Current Sensor (Three-Phase)  port_option=ee.enum.threePhasePort.composite
  PS-Simulink Converter : nesl_utility/PS-Simulink Converter  PhysicalDomain=network_engine_domain  SubClassName=ps_output  LeftPortType=input  RightPortType=output  PseudoPeriodic=off  Frequencies=[]  VectorFormat=1-D array  Unit=1  AffineConversion=off
  Park Transform : eeTransforms/Park Transform  AxisAlignment=D-axis  PowerInvariant=off
  ~1 : PMIOPort  Side=Left
  ~2 : PMIOPort  Port=2  Side=Right
  Output : Outport
  wires:
  PS-Simulink Converter/1 -> Park Transform/1
  Park Transform/1 -> Output/1
  Input/1 -> Park Transform/2
  connections:
  Current Sensor/LConn1 -- ~1/RConn1
  PS-Simulink Converter/LConn1 -- Current Sensor/RConn1
  Current Sensor/RConn2 -- ~2/RConn1

== system FOC_sensored/Mjerenje struje4 ==
  Input : Inport
  Current Sensor : ee_lib/Sensors & Transducers/Current Sensor (Three-Phase)  port_option=ee.enum.threePhasePort.composite
  PS-Simulink Converter : nesl_utility/PS-Simulink Converter  PhysicalDomain=network_engine_domain  SubClassName=ps_output  LeftPortType=input  RightPortType=output  PseudoPeriodic=off  Frequencies=[]  VectorFormat=1-D array  Unit=1  AffineConversion=off
  Park Transform : eeTransforms/Park Transform  AxisAlignment=D-axis  PowerInvariant=off
  ~1 : PMIOPort  Side=Left
  ~2 : PMIOPort  Port=2  Side=Right
  Output : Outport
  wires:
  PS-Simulink Converter/1 -> Park Transform/1
  Park Transform/1 -> Output/1
  Input/1 -> Park Transform/2
  connections:
  Current Sensor/LConn1 -- ~1/RConn1
  PS-Simulink Converter/LConn1 -- Current Sensor/RConn1
  Current Sensor/RConn2 -- ~2/RConn1

== system FOC_sensored/Mjerenje struje5 ==
  Input : Inport
  Current Sensor : ee_lib/Sensors & Transducers/Current Sensor (Three-Phase)  port_option=ee.enum.threePhasePort.composite
  PS-Simulink Converter : nesl_utility/PS-Simulink Converter  PhysicalDomain=network_engine_domain  SubClassName=ps_output  LeftPortType=input  RightPortType=output  PseudoPeriodic=off  Frequencies=[]  VectorFormat=1-D array  Unit=1  AffineConversion=off
  Park Transform : eeTransforms/Park Transform  AxisAlignment=D-axis  PowerInvariant=off
  ~1 : PMIOPort  Side=Left
  ~2 : PMIOPort  Port=2  Side=Right
  Output : Outport
  wires:
  PS-Simulink Converter/1 -> Park Transform/1
  Park Transform/1 -> Output/1
  Input/1 -> Park Transform/2
  connections:
  Current Sensor/LConn1 -- ~1/RConn1
  PS-Simulink Converter/LConn1 -- Current Sensor/RConn1
  Current Sensor/RConn2 -- ~2/RConn1

== system FOC_sensored/Mjerenje struje7 ==
  Input : Inport
  Current Sensor : ee_lib/Sensors & Transducers/Current Sensor (Three-Phase)  port_option=ee.enum.threePhasePort.composite
  PS-Simulink Converter : nesl_utility/PS-Simulink Converter  PhysicalDomain=network_engine_domain  SubClassName=ps_output  LeftPortType=input  RightPortType=output  PseudoPeriodic=off  Frequencies=[]  VectorFormat=1-D array  Unit=1  AffineConversion=off
  Park Transform : eeTransforms/Park Transform  AxisAlignment=D-axis  PowerInvariant=off
  ~1 : PMIOPort  Side=Left
  ~2 : PMIOPort  Port=2  Side=Right
  Output : Outport
  wires:
  PS-Simulink Converter/1 -> Park Transform/1
  Park Transform/1 -> Output/1
  Input/1 -> Park Transform/2
  connections:
  Current Sensor/LConn1 -- ~1/RConn1
  PS-Simulink Converter/LConn1 -- Current Sensor/RConn1
  Current Sensor/RConn2 -- ~2/RConn1

== system FOC_sensored/PWM inverter1 ==
  ud_ref : Inport
  uq_ref : Inport  Port=2
  theta_e_mj : Inport  Port=3
  Constant1 : Constant  Value=0  SampleTime=-1
  Gain : Gain
  Gain1 : Gain
  Mux2 : Mux  Inputs=2
  Mux3 : Mux  Inputs=2
  dq->abc : eeTransforms/Inverse Park Transform  AxisAlignment=D-axis  PowerInvariant=off
  u_abc* : Outport  VectorParamsAs1DForOutWhenUnconnected=off
  wires:
  Constant1/1 -> Mux2/2
  Mux2/1 -> dq->abc/1
  Mux3/1 -> Mux2/1
  theta_e_mj/1 -> dq->abc/2
  ud_ref/1 -> Gain/1
  uq_ref/1 -> Gain1/1
  Gain/1 -> Mux3/1
  Gain1/1 -> Mux3/2
  dq->abc/1 -> u_abc*/1

== system FOC_sensored/PWM inverter2 ==
  ud_ref : Inport
  uq_ref : Inport  Port=2
  theta_e_mj : Inport  Port=3
  Constant1 : Constant  Value=0  SampleTime=-1
  Gain : Gain
  Gain1 : Gain
  Mux2 : Mux  Inputs=2
  Mux3 : Mux  Inputs=2
  Zero-Order Hold1 : ZeroOrderHold  SampleTime=Ts_current
  dq->abc : eeTransforms/Inverse Park Transform  AxisAlignment=D-axis  PowerInvariant=off
  u_abc* : Outport  VectorParamsAs1DForOutWhenUnconnected=off
  wires:
  Constant1/1 -> Mux2/2
  Mux2/1 -> dq->abc/1
  Mux3/1 -> Mux2/1
  theta_e_mj/1 -> dq->abc/2
  dq->abc/1 -> Zero-Order Hold1/1
  ud_ref/1 -> Gain/1
  uq_ref/1 -> Gain1/1
  Gain/1 -> Mux3/1
  Gain1/1 -> Mux3/2
  Zero-Order Hold1/1 -> u_abc*/1

== system FOC_sensored/PWM inverter3 ==
  ud_ref : Inport
  uq_ref : Inport  Port=2
  theta_e_mj : Inport  Port=3
  Constant1 : Constant  Value=0  SampleTime=-1
  Gain : Gain
  Gain1 : Gain
  Mux2 : Mux  Inputs=2
  Mux3 : Mux  Inputs=2
  Zero-Order Hold1 : ZeroOrderHold  SampleTime=Ts_current
  dq->abc : eeTransforms/Inverse Park Transform  AxisAlignment=D-axis  PowerInvariant=off
  u_abc* : Outport  VectorParamsAs1DForOutWhenUnconnected=off
  wires:
  Constant1/1 -> Mux2/2
  Mux2/1 -> dq->abc/1
  Mux3/1 -> Mux2/1
  theta_e_mj/1 -> dq->abc/2
  dq->abc/1 -> Zero-Order Hold1/1
  ud_ref/1 -> Gain/1
  uq_ref/1 -> Gain1/1
  Gain/1 -> Mux3/1
  Gain1/1 -> Mux3/2
  Zero-Order Hold1/1 -> u_abc*/1

== system FOC_sensored/PWM inverter5 ==
  ud_ref : Inport
  uq_ref : Inport  Port=2
  theta_e_mj : Inport  Port=3
  Constant1 : Constant  Value=0  SampleTime=-1
  Gain : Gain
  Gain1 : Gain
  Mux2 : Mux  Inputs=2
  Mux3 : Mux  Inputs=2
  Zero-Order Hold1 : ZeroOrderHold  SampleTime=Ts_current
  dq->abc : eeTransforms/Inverse Park Transform  AxisAlignment=D-axis  PowerInvariant=off
  u_abc* : Outport  VectorParamsAs1DForOutWhenUnconnected=off
  wires:
  Constant1/1 -> Mux2/2
  Mux2/1 -> dq->abc/1
  Mux3/1 -> Mux2/1
  theta_e_mj/1 -> dq->abc/2
  dq->abc/1 -> Zero-Order Hold1/1
  ud_ref/1 -> Gain/1
  uq_ref/1 -> Gain1/1
  Gain/1 -> Mux3/1
  Gain1/1 -> Mux3/2
  Zero-Order Hold1/1 -> u_abc*/1

== system FOC_sensored/PWM inverter6 ==
  ud_ref : Inport
  uq_ref : Inport  Port=2
  theta_e_mj : Inport  Port=3
  Constant1 : Constant  Value=0  SampleTime=-1
  Gain : Gain
  Gain1 : Gain
  Mux2 : Mux  Inputs=2
  Mux3 : Mux  Inputs=2
  Zero-Order Hold1 : ZeroOrderHold  SampleTime=Ts_current
  dq->abc : eeTransforms/Inverse Park Transform  AxisAlignment=D-axis  PowerInvariant=off
  u_abc* : Outport  VectorParamsAs1DForOutWhenUnconnected=off
  wires:
  Constant1/1 -> Mux2/2
  Mux2/1 -> dq->abc/1
  Mux3/1 -> Mux2/1
  theta_e_mj/1 -> dq->abc/2
  dq->abc/1 -> Zero-Order Hold1/1
  ud_ref/1 -> Gain/1
  uq_ref/1 -> Gain1/1
  Gain/1 -> Mux3/1
  Gain1/1 -> Mux3/2
  Zero-Order Hold1/1 -> u_abc*/1

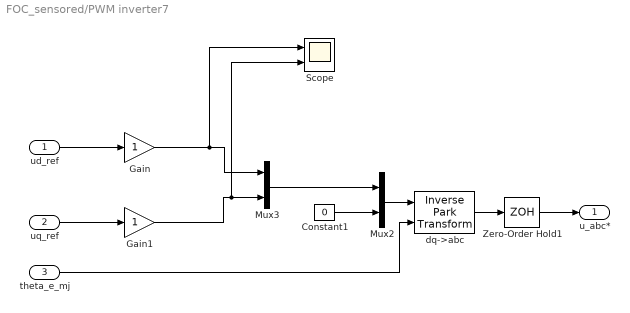
== system FOC_sensored/PWM inverter7 ==
  ud_ref : Inport
  uq_ref : Inport  Port=2
  theta_e_mj : Inport  Port=3
  Constant1 : Constant  Value=0  SampleTime=-1
  Gain : Gain
  Gain1 : Gain
  Mux2 : Mux  Inputs=2
  Mux3 : Mux  Inputs=2
  Scope : Scope  NumInputPorts=2
      settings: ActiveDisplayYMinimum=-5.00439749396322  ActiveDisplayYMaximum=16.069405098335697
  Zero-Order Hold1 : ZeroOrderHold  SampleTime=Ts_current
  dq->abc : eeTransforms/Inverse Park Transform  AxisAlignment=D-axis  PowerInvariant=off
  u_abc* : Outport  VectorParamsAs1DForOutWhenUnconnected=off
  wires:
  Constant1/1 -> Mux2/2
  Mux2/1 -> dq->abc/1
  Mux3/1 -> Mux2/1
  theta_e_mj/1 -> dq->abc/2
  dq->abc/1 -> Zero-Order Hold1/1
  ud_ref/1 -> Gain/1
  uq_ref/1 -> Gain1/1
  Gain/1 -> Scope/1, Mux3/1
  Gain1/1 -> Scope/2, Mux3/2
  Zero-Order Hold1/1 -> u_abc*/1

== matlab function FOC_sensored/Low-Pass Filter Current ==
  data: x input; y output; y_prev input; y_prev_out output; x_prev input; x_prev_out output; fc input; TS input
function [y, y_prev_out, x_prev_out] = fcn(x, y_prev, x_prev, fc, TS)



%% Convert to rad/s
omega_c = 2 * pi * fc;

%% Tustin coefficients
b =  omega_c / (2/TS + omega_c);
a = (omega_c - 2/TS) / (2/TS + omega_c);

%% Output
y = b * (x + x_prev) - a * y_prev;

%% State outputs — two separate scalars
y_prev_out = y;
x_prev_out = x;

end

== matlab function FOC_sensored/Low-Pass Filter Speed Ref ==
  data: x input; y output; y_prev input; y_prev_out output; x_prev input; x_prev_out output; fc input; TS input
function [y, y_prev_out, x_prev_out] = fcn(x, y_prev, x_prev, fc, TS)

%% Convert to rad/s
omega_c = 2 * pi * fc;

%% Tustin coefficients
b =  omega_c / (2/TS + omega_c);
a = (omega_c - 2/TS) / (2/TS + omega_c);

%% Output
y = b * (x + x_prev) - a * y_prev;

%% State outputs — two separate scalars
y_prev_out = y;
x_prev_out = x;

end

== matlab function FOC_sensored/Encoder ==
  data: angle input; theta_e output; omega_e output; angle_prev input; q_angle output; N input; dt input; pole_pairs input
function [theta_e, omega_e, q_angle] = fcn(angle, angle_prev, N, dt, pole_pairs)

%% Quantize current angle (simulate encoder resolution)
raw_count   = angle * (N / (2*pi));
counts      = floor(raw_count + 0.5);
q_angle     = counts * (2*pi / N);

%% Quantize previous angle the same way
raw_count_prev = angle_prev * (N / (2*pi));
counts_prev    = floor(raw_count_prev + 0.5);
q_angle_prev   = counts_prev * (2*pi / N);

%% Mechanical angular velocity (handle wrap-around)
delta = q_angle - q_angle_prev;

% Unwrap: if jump > pi, crossed zero boundary
if delta > pi
    delta = delta - 2*pi;
elseif delta < -pi
    delta = delta + 2*pi;
end

omega_m = delta / dt;       % mechanical rad/s

%% Convert to electrical quantities
theta_e = mod(q_angle, 2*pi);   % electrical angle [0, 2pi]
omega_e = omega_m;               % electrical rad/s

end

== matlab function FOC_sensored/Diskretni regulatori struje5/PI-controller ==
  data: error_id input; error_iq input; id input; iq input; we_prev input; vd output; vq output; vd_state_in input; vq_state_in input; error_id_prev input; error_iq_prev input; vd_state_out output; vq_state_out output; error_id_out output; error_iq_out output; ff_id_prev input; ff_iq_prev input; ff_id_out output; ff_iq_out output; K_P_current input; K_I_current input; TS input; L_Q input; L_D input; PHI_PM input; CURRENT_CONTROL_LIMIT input
function [vd, vq, vd_state_out, vq_state_out, ...
          error_id_out, error_iq_out, ff_id_out, ff_iq_out] = ...
          fcn(error_id, error_iq, id, iq, we_prev, ...
              vd_state_in, vq_state_in, ...
              error_id_prev, error_iq_prev, ...
              ff_id_prev, ff_iq_prev, K_P_current, K_I_current, TS, L_Q, L_D, PHI_PM, CURRENT_CONTROL_LIMIT)


%% Feedforward — using delayed we to break algebraic loop
ff_id = -iq * L_Q * we_prev;
ff_iq =  id * L_D * we_prev + PHI_PM * we_prev;

%% Tustin PI + FF delta
vd_ = vd_state_in ...
    + K_P_current * (error_id - error_id_prev) ...
    + K_I_current * (TS / 2) * (error_id + error_id_prev) ...
    + (ff_id - ff_id_prev);

vq_ = vq_state_in ...
    + K_P_current * (error_iq - error_iq_prev) ...
    + K_I_current * (TS / 2) * (error_iq + error_iq_prev) ...
    + (ff_iq - ff_iq_prev);

%% Circle clamp
voltage_magnitude = sqrt(vd_^2 + vq_^2);
if voltage_magnitude > CURRENT_CONTROL_LIMIT
    scale = CURRENT_CONTROL_LIMIT / voltage_magnitude;
    vd = vd_ * scale;
    vq = vq_ * scale;
else
    vd = vd_;
    vq = vq_;
end

%% State outputs
vd_state_out = vd;
vq_state_out = vq;
error_id_out = error_id;
error_iq_out = error_iq;
ff_id_out    = ff_id;      % → Unit Delay → ff_id_prev
ff_iq_out    = ff_iq;      % → Unit Delay → ff_iq_prev

end

== matlab function FOC_sensored/Diskretni regulator brzine5/PI-speed_controller ==
  data: speed_ref input; is_ref output; speed input; error_prev input; integrator_state input; error_out output; vd_state_out output; speed_ref_sat output; MAX_RPM input; K_P_speed input; K_I_speed input; TS input; IS_REF_LIMIT input
function [is_ref, error_out, vd_state_out,speed_ref_sat] = ...
          fcn(speed_ref, speed, error_prev, integrator_state, MAX_RPM, K_P_speed, K_I_speed, TS, IS_REF_LIMIT)



%% Saturate speed reference
if speed_ref > MAX_RPM
    speed_ref_sat = MAX_RPM;
elseif speed_ref < -MAX_RPM
    speed_ref_sat = -MAX_RPM;
else
    speed_ref_sat = speed_ref;
end

%% Error
error_curr = speed_ref_sat - speed;

%% --- Tustin (bilinear) PI ---
%
%  Continuous PI:   u(s) = Kp * e(s) + Ki/s * e(s)
%
%  Tustin:  integrator  1/s  ->  T/2 * (z+1)/(z-1)
%
%  Incremental form:
%    u[k] = u[k-1] + Kp*(e[k] - e[k-1]) + Ki*T/2*(e[k] + e[k-1])

is_ref_raw = integrator_state ...
           + K_P_speed * (error_curr - error_prev) ...
           + K_I_speed * (TS / 2.0) * (error_curr + error_prev);

%% Saturate is_ref (anti-windup: clamp before feeding state back)
if is_ref_raw > IS_REF_LIMIT
    is_ref = IS_REF_LIMIT;
elseif is_ref_raw < -IS_REF_LIMIT
    is_ref = -IS_REF_LIMIT;
else
    is_ref = is_ref_raw;
end

%% State outputs → Unit Delays → next step inputs
error_out      = error_curr;   % → Unit Delay → error_prev
vd_state_out   = is_ref;       % → Unit Delay → integrator_state (clamped = anti-windup)

end

== matlab function FOC_sensored/Low-Pass Filter Speed ==
  data: x input; y output; y_prev input; y_prev_out output; x_prev input; x_prev_out output; fc input; TS input
function [y, y_prev_out, x_prev_out] = fcn(x, y_prev, x_prev, fc, TS)


%% Convert to rad/s
omega_c = 2 * pi * fc;

%% Tustin coefficients
b =  omega_c / (2/TS + omega_c);
a = (omega_c - 2/TS) / (2/TS + omega_c);

%% Output
y = b * (x + x_prev) - a * y_prev;

%% State outputs — two separate scalars
y_prev_out = y;
x_prev_out = x;

end
